simulink model "StateObserv_StateFeedback"  (R2024b)
settings: Solver=VariableStepAuto  StartTime=0.0  StopTime=10  RelTol=1e-3
values from neighbouring files (symbols this model uses):
  A = [0   1          0               0 ... (first row only)    [main.m]
  B = [0; 1/M; 0; b/(M*L)]    [main.m]
  C = [1 0 0 0 ... (first row only)    [main.m]
  K = lqr(A, B, Q, R)    [main.m]
  Lc = place(A', C', observer_poles)'    [main.m]
settings Model: Creator=98912  LastModifiedBy=98912

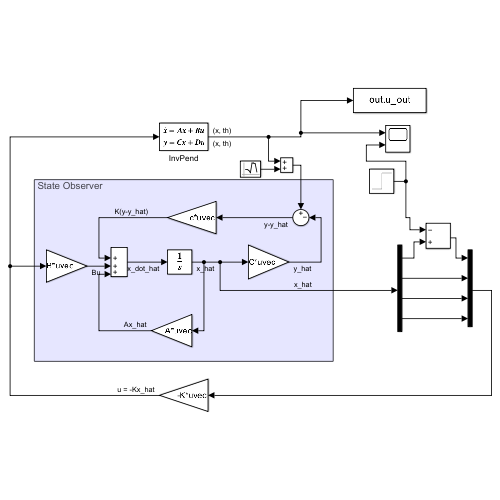
[thumbnail: Simulink's stored preview of the top-level diagram]
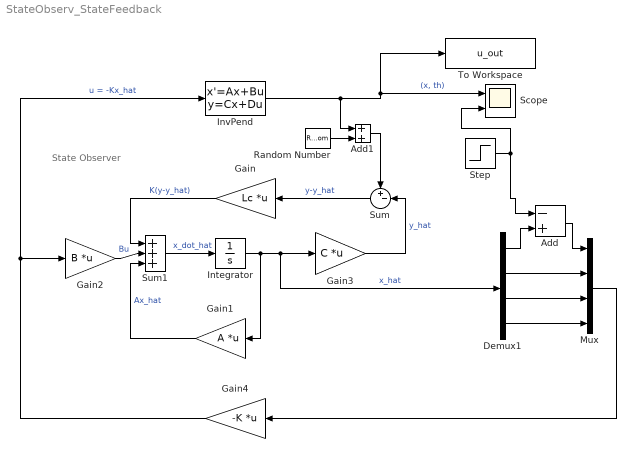
== system StateObserv_StateFeedback ==
  note: State Observer
  Add : Sum  Inputs=-+
  Add1 : Sum
  Demux1 : Demux
  Gain : Gain  Gain=Lc  Multiplication=Matrix(K*u) (u vector)
  Gain1 : Gain  Gain=A  Multiplication=Matrix(K*u) (u vector)
  Gain2 : Gain  Gain=B  Multiplication=Matrix(K*u) (u vector)
  Gain3 : Gain  Gain=C  Multiplication=Matrix(K*u) (u vector)
  Gain4 : Gain  Gain=-K  Multiplication=Matrix(K*u) (u vector)
  Integrator : Integrator  InitialCondition=[0;0;0.2;0]
  InvPend : StateSpace  A=A  B=B  C=C  D=[0; 0]  InitialCondition=[0;0;0.2;0]
  Mux : Mux
  Random Number : RandomNumber  Variance=0.00001  SampleTime=0.1
  Scope : Scope  NumInputPorts=2
  Step : Step  Time=2  After=2  SampleTime=0
  Sum : Sum  Inputs=+-|
  Sum1 : Sum  Inputs=|+++
  To Workspace : ToWorkspace  VariableName=u_out  SaveFormat=Timeseries  SampleTime=-1
  wires:
  Demux1/3 -> Mux/3
  Gain4/1 -> Gain2/1, InvPend/1  "u = -Kx_hat"
  Demux1/4 -> Mux/4
  Demux1/1 -> Add/2
  Mux/1 -> Gain4/1
  InvPend/1 -> Add1/1, Scope/1, To Workspace/1  "(x, th)"
  Demux1/2 -> Mux/2
  Gain1/1 -> Sum1/3  "Ax_hat"
  Gain2/1 -> Sum1/2  "Bu"
  Sum/1 -> Gain/1  "y-y_hat"
  Sum1/1 -> Integrator/1  "x_dot_hat"
  Gain3/1 -> Sum/2  "y_hat"
  Integrator/1 -> Demux1/1, Gain3/1, Gain1/1  "x_hat"
  Gain/1 -> Sum1/1  "K(y-y_hat)"
  Step/1 -> Add/1, Scope/2
  Add/1 -> Mux/1
  Random Number/1 -> Add1/2
  Add1/1 -> Sum/1
